simulink model "CPG_2021a"  (R2022a)
settings: Solver=VariableStepAuto  StartTime=0.0  StopTime=10  RelTol=1e-3
values from neighbouring files (symbols this model uses):
  ar = 2    [Snake5animal.m]    (also in animal.m; parameters.m)
  ax = 2    [Snake5animal.m]    (also in animal.m; parameters.m)
  N = 5    [Snake5animal.m]
  omega = ones(1,N)*0.6*pi    [Snake5animal.m]    (also in animal.m = ones(3,3)*2; parameters.m = ones(3,3)*0.5)
  omega1 = 0.6*pi    (= 1.88495559215)    [animal.m]    (also in parameters.m = 0)
  omega2 = 0.6*pi    (= 1.88495559215)    [animal.m]    (also in parameters.m = 0)
  omega3 = 0.6*pi    (= 1.88495559215)    [animal.m]    (also in parameters.m = 0)
  phi = ones(3,3)*PHI    [animal.m]    (also in parameters.m = zeros(3,3))
  R1 = R1    [animal.m]    (also in parameters.m = 4)
  R2 = R2    [animal.m]    (also in parameters.m = 4)
  R3 = R3    [animal.m]    (also in parameters.m = 4)
  X = zeros(1,N)    [Snake5animal.m]
  X1 = 0    [animal.m]    (also in parameters.m)
  X2 = 0    [animal.m]    (also in parameters.m)
  X3 = 0    [animal.m]    (also in parameters.m)
undefined symbols (not defined in the file or in its folder): Y, Z
libraries: sm_lib x23, nesl_utility x6
(part 2 of 2)

== system CPG_2021a/Subsystem/Subsystem3/Subsystem2/Subsystem3/Subsystem1 ==
  psij : Inport
  psii : Inport  Port=2
  phiij : Inport  Port=3
  Add1 : Sum  Inputs=+--
  Trigonometric Function1 : Trigonometry
  Out1 : Outport
  wires:
  psij/1 -> Add1/1
  phiij/1 -> Add1/3
  psii/1 -> Add1/2
  Add1/1 -> Trigonometric Function1/1
  Trigonometric Function1/1 -> Out1/1

== system CPG_2021a/Subsystem/Subsystem3/Subsystem2/Subsystem3/Subsystem2 ==
  psij : Inport
  psii : Inport  Port=2
  phiij : Inport  Port=3
  Add1 : Sum  Inputs=+--
  Trigonometric Function1 : Trigonometry
  Out1 : Outport
  wires:
  psij/1 -> Add1/1
  phiij/1 -> Add1/3
  psii/1 -> Add1/2
  Add1/1 -> Trigonometric Function1/1
  Trigonometric Function1/1 -> Out1/1
